simulink model "buck"  (R2014a)
settings: Solver=ode45  StartTime=0.0  StopTime=0.05  RelTol=1e-3
libraries: powerlib x9, simulink x1
settings Model: Creator=Zaid  LastModifiedBy=Zaid

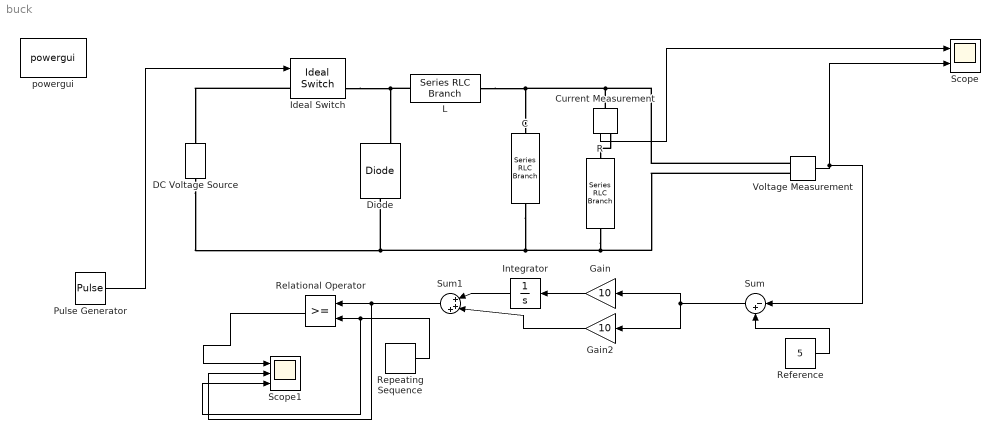
== system buck ==
  C : powerlib/Elements/Series RLC Branch  LConnTagsString=__new0  RConnTagsString=__new0  BranchType=C  Resistance=1  Inductance=327e-6  SetiL0=off  InitialCurrent=0  Capacitance=750e-9  Setx0=off  InitialVoltage=0  Measurements=None
  Current Measurement : powerlib/Measurements/Current Measurement  PhasorSimulation=off  OutputType=Complex  PSBequivalent=0
  DC Voltage Source : powerlib/Electrical Sources/DC Voltage Source  Amplitude=14.5  Measurements=None
  Diode : powerlib/Power Electronics/Diode  Ron=0.001  Lon=0  Vf=0  IC=0  UseSnubber=off  Rs=500  Cs=250e-9  Measurements=on
  Gain : Gain  Gain=10
  Gain2 : Gain  Gain=10
  Ideal Switch : powerlib/Power Electronics/Ideal Switch  Ron=0.001  Lon=0  IC=0  Rs=1e5  Cs=inf  Measurements=on
  Integrator : Integrator
  L : powerlib/Elements/Series RLC Branch  LConnTagsString=__new0  RConnTagsString=__new0  BranchType=L  Resistance=1  Inductance=109.195e-6  SetiL0=off  InitialCurrent=0  Capacitance=1e-6  Setx0=off  InitialVoltage=0  Measurements=None
  Pulse Generator : DiscretePulseGenerator  PulseType=Time based  Amplitude=10  Period=1/100000  PulseWidth=34.48
  R : powerlib/Elements/Series RLC Branch  LConnTagsString=__new0  RConnTagsString=__new0  BranchType=R  Resistance=5  Inductance=327e-6  SetiL0=off  InitialCurrent=0  Capacitance=1.25e-8  Setx0=off  InitialVoltage=0  Measurements=None
  Reference : Constant  Value=5
  Relational Operator : RelationalOperator  OutDataTypeStr=boolean  ZeroCross=off
  Repeating Sequence : simulink/Sources/Repeating Sequence  rep_seq_t=[0 1/1000000]  rep_seq_y=[0 50]
  Scope : Scope  NumInputPorts=2
      settings: YMin=0.83~4.15  YMax=0.9~4.5
  Scope1 : Scope  NumInputPorts=3
      settings: YMin=0.000499975~0.00249975~-5  YMax=0.00050055~0.00250275~5
  Sum : Sum  Inputs=|-+
  Sum1 : Sum  Inputs=|+++
  Voltage Measurement : powerlib/Measurements/Voltage Measurement  PhasorSimulation=off  OutputType=Complex  PSBequivalent=0
  powergui : powerlib/powergui  Priority=1  SimulationMode=Continuous  SolverType=Tustin  SampleTime=50e-6  frequency=60  SPID=off  DisableSnubberDevices=off  DisableRonSwitches=off  DisableVfSwitches=off  SwTol=0  Interpol=off  DisplayEquations=off  Ts=0  methode=off  frequencyindice=0  Pbase=100e6  ErrMax=1e-4  Iterations=50  UnitsV=kV  UnitsW=MW  FunctionMessages=off  echomessages=off  HookPort=off  EnableUseOfTLC=off  x0status=blocks  RestoreLinks=warning  ResistiveCurrentMeasurement=off  Frange=[0:2:500]  Ylog=off  Xlog=on  ShowGrid=off  save=off  variable=ZData  structure=0  ZoomFFT=off  StartTime=0.0  cycles=1  DisplayStyle=1  fundamental=60  FreqAxis=off  MaxFrequency=1000  frequencyindicesteady=1  RmsSteady=1  display=off
  wires:
  Current Measurement/1 -> Scope/1
  Voltage Measurement/1 -> Sum/1, Scope/2
  Reference/1 -> Sum/2
  Sum/1 -> Gain2/1, Gain/1
  Gain/1 -> Integrator/1
  Integrator/1 -> Sum1/1
  Gain2/1 -> Sum1/2
  Sum1/1 -> Scope1/2, Relational Operator/1
  Repeating Sequence/1 -> Scope1/3, Relational Operator/2
  Relational Operator/1 -> Scope1/1
  Pulse Generator/1 -> Ideal Switch/1
  connections:
  Ideal Switch/LConn1 -- DC Voltage Source/RConn1
  L/RConn1 -- Voltage Measurement/LConn1 -- Current Measurement/LConn1 -- C/LConn1
  L/LConn1 -- Ideal Switch/RConn1 -- Diode/RConn1
  C/RConn1 -- R/RConn1 -- Voltage Measurement/LConn2 -- Diode/LConn1 -- DC Voltage Source/LConn1
  Current Measurement/RConn1 -- R/LConn1
